simulink model "Example_4_Open"  (Simulink 8.3)
settings: Solver=ode45  StartTime=0.0  StopTime=40  RelTol=1e-3
settings Model: Creator=Li Jinghao  LastModifiedBy=Li Jinghao
settings DataIOCC: SignalLoggingSaveFormat=Dataset
settings DebuggingCC: UnderspecifiedInitializationDetection=Simplified  StateNameClashWarn=none
settings GRTTargetCC: CombineOutputUpdateFcns=on  GRTInterface=off

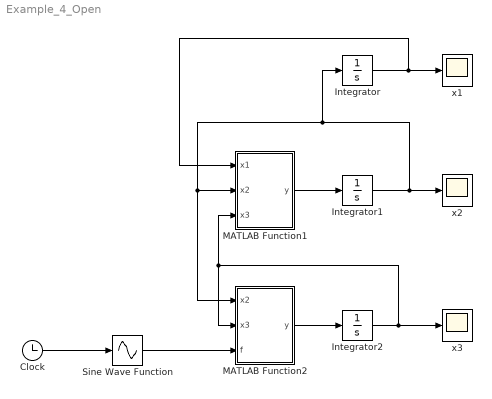
== system Example_4_Open ==
  Clock : Clock
  Integrator : Integrator  InitialCondition=pi/8
  Integrator1 : Integrator
  Integrator2 : Integrator  InitialCondition=0.8
  MATLAB Function1 : MATLAB Function  TreatAsAtomicUnit=on
  MATLAB Function2 : MATLAB Function  TreatAsAtomicUnit=on
  Sine Wave Function : Sin  TimeSource=Use external signal  Bias=1  SampleTime=0
  x1 : Scope
      settings: SaveName=x1
  x2 : Scope
      settings: SaveName=x2
  x3 : Scope
      settings: SaveName=x3
  wires:
  Integrator2/1 -> MATLAB Function2/2(x3), MATLAB Function1/3(x3), x3/1
  Integrator1/1 -> Integrator/1, MATLAB Function2/1(x2), MATLAB Function1/2(x2), x2/1
  Integrator/1 -> MATLAB Function1/1(x1), x1/1
  MATLAB Function1/1(y) -> Integrator1/1
  MATLAB Function2/1(y) -> Integrator2/1
  Clock/1 -> Sine Wave Function/1
  Sine Wave Function/1 -> MATLAB Function2/3(f)

== matlab function MATLAB Function1 ==
  data: x1 input double; y output double; x2 input double; x3 input double
function y = fcn(x1,x2,x3)
%#codegen

Jm=0.126*10^-3;
alpha=0.001;
l=0.2;
m=0.1;
km=0.0446;
g=9.81;

y = 1/(Jm+m*l*l)*(-m*g*l*sin(x1)-alpha*x2+km*x3);

== matlab function MATLAB Function2 ==
  data: x2 input double; y output double; x3 input double; f input double
function y = fcn(x2,x3,f)
%#codegen

R=0.1;
L=92;
ke=0.076;

y = 1/L*(-ke*x2-R*x3+f);
